simulink model "Demo"  (Simulink 6.5)
settings: Solver=ode45  StartTime=0.0  StopTime=10.0  RelTol=1e-3
settings Model: Creator=suarezjl  LastModifiedBy=suarezjl
settings DataIOCC: SignalLoggingName=sigsOut
settings DebuggingCC: SolverPrmCheckMsg=none  MultiTaskDSMMsg=warning  MultiTaskCondExecSysMsg=none  StrictBusMsg=None
settings HardwareCC: TargetUnknown=on
settings RTWCC: IncludeERTFirstTime=on

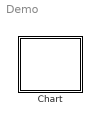
== system Demo ==
  Chart : Stateflow chart

== stateflow chart Chart ==
  state Start Cameras State Machine in Sally
    \\Sally\RightReachDemo\HeadModule\LeftCameraAgent\StateMachine.LoadSM()
    \\Sally\RightReachDemo\HeadModule\LeftCameraAgent\StateMachine.Start()
    \\Sally\RightReachDemo\HeadModule\RightCameraAgent\StateMachine.LoadSM()
    \\Sally\RightReachDemo\HeadModule\RightCameraAgent\StateMachine.Start()
    \\Sally\RightReachDemo\HeadModule\RightCameraAgent\StateMachine.Wait(50)
  state Start Head
    \\Sally\RightReachDemo\HeadModule\HeadAgent\StateMachine.LoadSM()
    \\Sally\RightReachDemo\HeadModule\HeadAgent\StateMachine.Start()
    \\Sally\RightReachDemo\HeadModule\HeadAgent\StateMachine.Wait(50)
  state Stop
    \\Hungerforce\RightReachDemo\RightArm\StateMachine.Stop()
    \\Hungerforce\RightReachDemo\RightTrajectoryAgent\StateMachine.Stop()
    \\Hungerforce\RightReachDemo\RightArm\SampleIndPressure.Reset()
    \\Sally\RightReachDemo\HeadModule\LeftCameraAgent\StateMachine.Stop()
    \\Sally\RightReachDemo\HeadModule\RightCameraAgent\StateMachine.Stop()
    \\Sally\RightReachDemo\HeadModule\HeadAgent\StateMachine.Stop()
    \\Sally\RightReachDemo\HeadModule\HeadAgent\EyeMotionControl.Initial()
  state Start Arm
    \\Hungerforce\RightReachDemo\RightArm\StateMachine.LoadSM()
    \\Hungerforce\RightReachDemo\RightArm\StateMachine.Start()
    \\Hungerforce\RightReachDemo\RightArm\StateMachine.Wait(1000)
  (default) -> Start Arm : Start
  Start Cameras State Machine in Sally -> Start Head : Always
  Start Head -> Stop : Signal="Stop"
  Start Arm -> Start Cameras State Machine in Sally : Always
